simulink model "quat_rectify_test"  (R2018b)
settings: Solver=VariableStepAuto  StartTime=0.0  StopTime=10.0  RelTol=1e-3
libraries: vrlib x1, quat_rectify_lib x1
settings Model: Creator=Taylor  LastModifiedBy=Taylor

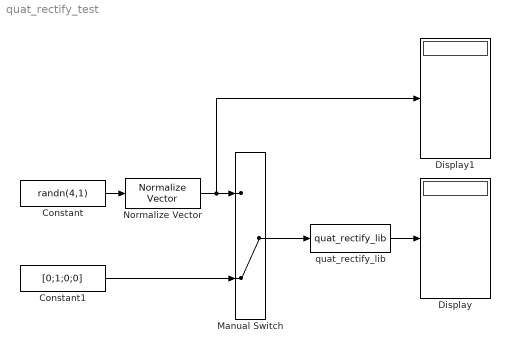
== system quat_rectify_test ==
  Constant : Constant  Value=randn(4,1)
  Constant1 : Constant  Value=[0;1;0;0]
  Display : Display
  Display1 : Display
  Manual Switch : ManualSwitch  CurrentSetting=0
  Normalize Vector : vrlib/Utilities/Normalize Vector  maxzero=0
      settings: SourceProductName=Simulink 3D Animation  SourceProductBaseCode=VR
  quat_rectify_lib : quat_rectify_lib/quat_rectify_lib
  wires:
  Constant/1 -> Normalize Vector/1
  Normalize Vector/1 -> Display1/1, Manual Switch/1
  Manual Switch/1 -> quat_rectify_lib/1
  Constant1/1 -> Manual Switch/2
  quat_rectify_lib/1 -> Display/1
